simulink model "akh_rev_project"  (R2020b)
settings: Solver=ode45  StartTime=0.0  StopTime=10  FixedStep=Ts_Power  RelTol=1e-3  AbsTol=1e-2
InitFcn:
  | Fnom = 50;        % Hz
  | 
  | Fc = 27*Fnom;   % (Hz)
  | Ts_Power = 1/(Fc*100);
  | Ts_Control = Ts_Power*10;
values from neighbouring files (symbols this model uses):
  Ts = 1/fs    (= 1e-05)    [PE_46.m]    (also in disc_sim.m = 1; mass_spring_damper_model.m = 0.1)
undefined symbols (not defined in the file or in its folder): D1, D11, Delta, DiscIntNeverNeededParam, j, magnitude
libraries: powerlib x146, powerlib_meascontrol x90, simulink x2, re_lib x1
(part 1 of 8)
Description:
  | The 'Model  initialization function' defined in the
  | 
  | Model Properties automatically sets the sample time
  | 
  | Ts to 50e-6 s
settings Model: FPTRunName=Active  ExtModeTrigMode=oneshot  ExtModeArmWhenConnect=off  ExtModeAutoUpdateStatusClock=off  Creator=MathWorks  LastModifiedBy=Dhanush Wagle
settings SolverCC: AutoScaleAbsTol=off
settings DataIOCC: SaveFormat=StructureWithTime  SignalLoggingSaveFormat=ModelDataLogs  SaveTime=off  ReturnWorkspaceOutputs=off  SignalLoggingName=sigsOut
settings OptimizationCC: BlockReduction=off  BooleanDataType=off  ExpressionDepthLimit=2147483647  InitFltsAndDblsToZero=on  LifeSpan=inf
settings DebuggingCC: SaveWithParameterizedLinksMsg=none  UnderspecifiedInitializationDetection=Classic  MergeDetectMultiDrivingBlocksExec=none  CheckExecutionContextPreStartOutputMsg=on  CheckExecutionContextRuntimeOutputMsg=on  SignalResolutionControl=TryResolveAllWithWarning  MultiTaskDSMMsg=warning  MultiTaskCondExecSysMsg=none  FcnCallInpInsideContextMsg=warning  UnconnectedInputMsg=none  UnconnectedOutputMsg=none  UnconnectedLineMsg=none  StateNameClashWarn=warning  SFUnexpectedBacktrackingDiag=warning  SFNoUnconditionalDefaultTransitionDiag=warning  SFExecutionAtInitializationDiag=none  ArithmeticOperatorsInVariantConditions=warning
settings HardwareCC: ProdBitPerPointer=32  ProdBitPerSizeT=32  ProdBitPerPtrDiffT=32  ProdLargestAtomicFloat=None  ProdIntDivRoundTo=Undefined  ProdEndianess=Unspecified  ProdWordSize=32  ProdHWDeviceType=32-bit Generic  TargetHWDeviceType=32-bit Generic  ProdEqTarget=off
settings ModelReferenceCC: PropagateSignalLabelsOutOfModel=off
settings SFSimCC: SimUseLocalCustomCode=off  CustomCodeUndefinedFunction=UseInterfaceOnly
settings RTWCC: RTWUseLocalCustomCode=off
settings CodeAppCC: StateflowObjectComments=on
settings GRTTargetCC: TargetFcnLib=ansi_tfl_tmw.mat  TargetLangStandard=C89/C90 (ANSI)  CombineOutputUpdateFcns=off  GRTInterface=on
settings ConfigComp: CovMetricSettings=dw  CovSaveCumulativeToWorkspaceVar=on  CovSaveSingleToWorkspaceVar=on  CovExternalEMLEnable=off  CovSFcnEnable=off
settings SimscapeCC: SimscapeNormalizeSystem=off

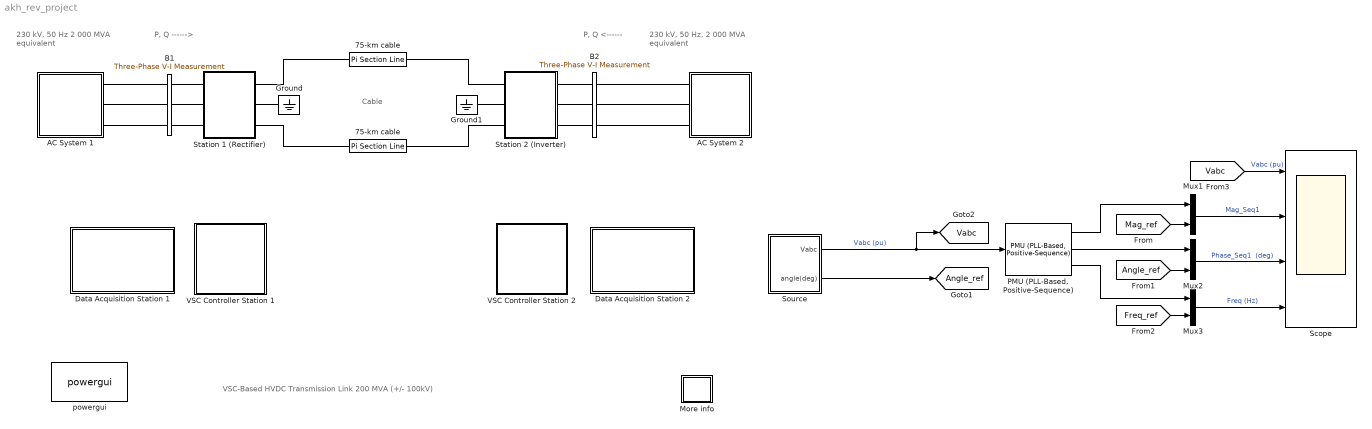
== system akh_rev_project ==
  note: VSC-Based HVDC Transmission Link 200 MVA (+/- 100kV)
  note: 230 kV, 50 Hz,
      | 2 000 MVA equivalent
  note: Cable
  note: P, Q
      | ------>
  note: P, Q
      | <------
  note: 230 kV, 50 Hz
      |  2 000 MVA equivalent
  75-km cable : powerlib/Elements/Pi Section Line  LConnTagsString=__new0  RConnTagsString=__new0  Phases=1  PiSections=2  Length=75  Frequency=Fnom  Resistance=1.3900e-002  Inductance=1.5900e-004  Capacitance=2.3100e-007  Measurements=None  Measurements2=None
      settings: AttributesFormatString=\n  SourceProductBaseCode=PS
  "75-km cable " : powerlib/Elements/Pi Section Line  LConnTagsString=__new0  RConnTagsString=__new0  Phases=1  PiSections=2  Length=75  Frequency=Fnom  Resistance=1.3900e-002  Inductance=1.5900e-004  Capacitance=2.3100e-007  Measurements=None  Measurements2=None
      settings: AttributesFormatString=\n  SourceProductBaseCode=PS
  AC System 1 : Subsystem
  AC System 2 : Subsystem
  B1 : powerlib/Measurements/Three-Phase V-I Measurement  VoltageMeasurement=phase-to-ground  SetLabelV=on  LabelV=Uabc_B1  Vpu=on  VpuLL=off  CurrentMeasurement=yes  SetLabelI=on  LabelI=Iabc_B1  Ipu=on  Pbase=200e6  Vbase=230e3  OutputType=Magnitude  PhasorSimulation=off  PSBequivalent=0
  B2 : powerlib/Measurements/Three-Phase V-I Measurement  VoltageMeasurement=phase-to-ground  SetLabelV=on  LabelV=Uabc_B2  Vpu=on  VpuLL=off  CurrentMeasurement=yes  SetLabelI=on  LabelI=Iabc_B2  Ipu=on  Pbase=200e6  Vbase=230e3  OutputType=Magnitude  PhasorSimulation=off  PSBequivalent=0
  Data Acquisition Station 1 : Subsystem
      mask Display: disp('Open this block\nto visualize\nrecorded signals')
  Data Acquisition Station 2 : Subsystem
      mask Display: disp('Open this block\nto visualize\nrecorded signals')
  Ground : powerlib/Elements/Ground  LConnTagsString=a
  Ground1 : powerlib/Elements/Ground  LConnTagsString=a
  More info : Subsystem
      settings: OpenFcn=showdemo(bdroot(gcb))
      mask Display: disp('?')
  Mux1 : Mux  Inputs=2
  Mux2 : Mux  Inputs=2
  Mux3 : Mux  Inputs=2
  "PMU (PLL-Based, Positive-Sequence)" : powerlib_meascontrol/Measurements/PMU (PLL-Based, Positive-Sequence)  nominalFrequency=60  samplingRate=64  reportingFactor=0.5
      settings: SourceProductBaseCode=PS
  Scope : Scope  NumInputPorts=4
  Source : Subsystem
  Station 1 (Rectifier) : Subsystem
  Station 2 (Inverter) : Subsystem
  VSC Controller Station 1 : Subsystem
      mask Display: disp('VSC\nPole Control')
  VSC Controller Station 2 : Subsystem
      mask Display: disp('VSC\nPole Control')
  powergui : powerlib/powergui  Priority=2  SimulationMode=Discrete  SampleTime=Ts_Power  frequency=60  Iterations=50  frequencyindice=60  Pbase=100e6  ErrMax=1e-4  UnitsV=kV  UnitsW=MW  buscounter=0  FunctionMessages=off  echomessages=off  EnableUseOfTLC=off  CurrentSourceSwitches=off  DisableSnubberDevices=off  DisableRonSwitches=off  DisableVfSwitches=off  DisplayEquations=off  AutomaticDiscreteSolvers=off  SolverType=Tustin/Backward Euler (TBE)  Interpol=off  ExternalGateDelay=off  methode=off  Ts=0  x0status=blocks  SPID=off  SwTol=0  HookPort=off  NonlinearTolerance=1e-4  nMaxIteration=100  ContinueOnMaxIteration=off  RestoreLinks=warning  ResistiveCurrentMeasurement=off  Frange=[0:2:500]  Ylog=off  Xlog=on  ShowGrid=off  save=off  variable=ZData  structure=res_fft  ZoomFFT=on  StartTime=1.5  cycles=2  DisplayStyle=1  fundamental=50  FreqAxis=off  MaxFrequency=3000  frequencyindicesteady=1  RmsSteady=1  display=off
  tag scope: Angle_ref=global, Vabc=global
  wires:
  [Mag_ref] -> Mux1/2
  Mux2/1 -> Scope/3  "Phase_Seq1  (deg)"
  Source/2(angle(deg)) -> [Angle_ref]
  "PMU (PLL-Based, Positive-Sequence)"/2 -> Mux2/1
  "PMU (PLL-Based, Positive-Sequence)"/3 -> Mux3/1
  [Vabc] -> Scope/1  "Vabc (pu)"
  [Angle_ref] -> Mux2/2
  [Freq_ref] -> Mux3/2
  Mux3/1 -> Scope/4  "Freq (Hz)"
  Mux1/1 -> Scope/2  "Mag_Seq1"
  "PMU (PLL-Based, Positive-Sequence)"/1 -> Mux1/1
  Source/1(Vabc) -> [Vabc], "PMU (PLL-Based, Positive-Sequence)"/1  "Vabc (pu)"
  connections:
  Station 1 (Rectifier)/LConn1 -- B1/RConn1
  B1/RConn2 -- Station 1 (Rectifier)/LConn2
  Station 1 (Rectifier)/LConn3 -- B1/RConn3
  "75-km cable "/LConn1 -- Station 1 (Rectifier)/RConn3
  75-km cable/RConn1 -- Station 2 (Inverter)/RConn1
  "75-km cable "/RConn1 -- Station 2 (Inverter)/RConn3
  B2/LConn1 -- AC System 2/RConn1
  Station 2 (Inverter)/LConn1 -- B2/RConn1
  Station 2 (Inverter)/LConn2 -- B2/RConn2
  Station 2 (Inverter)/LConn3 -- B2/RConn3
  B2/LConn2 -- AC System 2/RConn2
  B2/LConn3 -- AC System 2/RConn3
  Ground/LConn1 -- Station 1 (Rectifier)/RConn2
  Ground1/LConn1 -- Station 2 (Inverter)/RConn2
  AC System 1/RConn1 -- B1/LConn1
  AC System 1/RConn2 -- B1/LConn2
  AC System 1/RConn3 -- B1/LConn3
  Station 1 (Rectifier)/RConn1 -- 75-km cable/LConn1

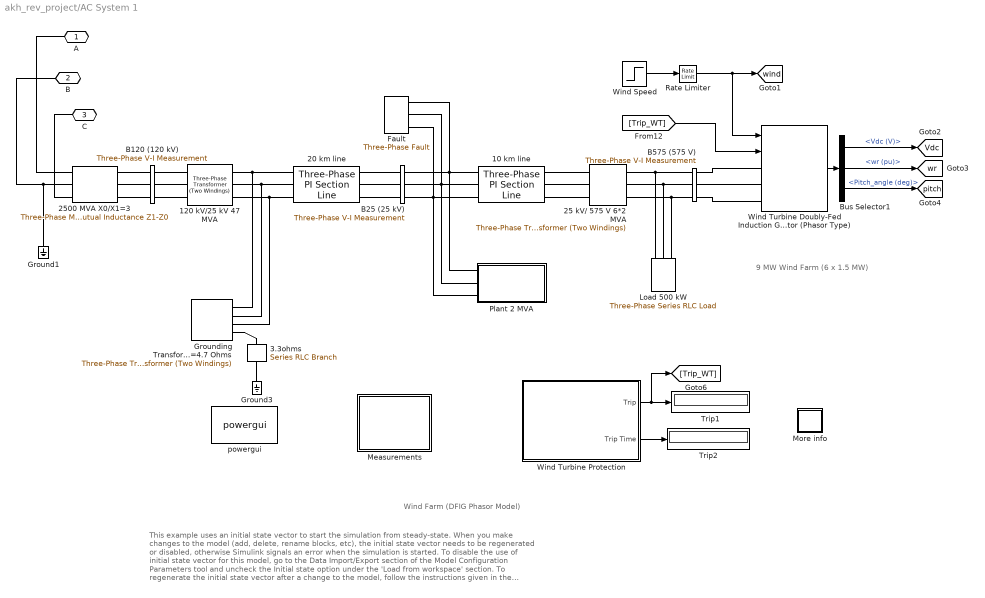
== system akh_rev_project/AC System 1 ==
  note: This example uses an initial state vector to start the simulation from steady-state. When you make changes to the model (add, delete, rename blocks, etc),
      | the initial state vector needs to be regenerated or disabled, otherwise Simulink signals an error when the simulation is started.
      | To disable the use of initial state vector for this model, go to the Data Import/Export section of the Model Configuration Parameters tool and uncheck the
      | Initial state option under the 'Load from workspace' section.
      | To regenerate the initial state vector after a change to the model, follow the instructions given in the initialization file for this model.
      | Type open('init_power_wind_dfig') at the matlab prompt to view this file.
  note: 9 MW Wind Farm
      | (6 x 1.5 MW)
  note: Wind Farm (DFIG Phasor Model)
  10 km line : powerlib/Elements/Three-Phase PI Section Line  LConnTagsString=a|b|c  RConnTagsString=A|B|C  Length=10  Frequency=60  Resistances=[0.1153 0.413]  Inductances=[1.05e-3 3.32e-3]  Capacitances=[11.33e-009 5.01e-009]
  120 kV/25 kV 47 MVA : powerlib/Elements/Three-Phase Transformer (Two Windings)  Winding1Connection=Yg  Winding2Connection=Delta (D1)  CoreType=Three single-phase transformers  SetSaturation=off  Hysteresis=off  DataFile='basic_model'  SetInitialFlux=off  Measurements=None  UNITS=pu  NominalPower=[47e6 60 ]  Winding1="[ 120e3  0.08/30   0.08 ]"  Winding2="[ 25e3  0.08/30  0.08]"  Rm=500  Lm=500  L0=0.5  Saturation="[ 0,0  ;  0.005,1.2  ;  1.0,1.4 ]"  InitialFluxes=[ 0.8 , -0.8 , 0.7 ]  BreakLoop=off  DiscreteSolver=Trapezoidal iterative  DataType=off  TransfoNumber=0
  20 km line : powerlib/Elements/Three-Phase PI Section Line  LConnTagsString=a|b|c  RConnTagsString=A|B|C  Length=20  Frequency=60  Resistances=[0.1153 0.413]  Inductances=[1.05e-3 3.32e-3]  Capacitances=[11.33e-009 5.01e-009]
  25 kV/ 575 V 6*2 MVA : powerlib/Elements/Three-Phase Transformer (Two Windings)  Winding1Connection=Yg  Winding2Connection=Delta (D1)  CoreType=Three single-phase transformers  SetSaturation=off  Hysteresis=off  DataFile='hysteresis'  SetInitialFlux=off  Measurements=None  UNITS=pu  NominalPower="[2e6*6  60]"  Winding1=[25e3 , 0.025/30 , 0.025]  Winding2=[ 575, 0.025/30 , 0.025]  Rm=500  Lm=inf  L0=0.5  Saturation=[ 0,0 ; 0.0024,1.2 ; 1.0,1.52 ]  InitialFluxes=[ 0.8 , -0.8 , 0.7 ]  BreakLoop=off  DiscreteSolver=Trapezoidal iterative  DataType=off  TransfoNumber=0
  2500 MVA X0/X1=3 : powerlib/Elements/Three-Phase Mutual Inductance Z1-Z0  LConnTagsString=a|b|c  RConnTagsString=A|B|C  PositiveSequence="[0.1  1.0/(2*pi*60)] *120e3^2/2500e6"  ZeroSequence="[0.3  3.0/(2*pi*60)] *120e3^2/2500e6"
      settings: SourceProductBaseCode=PS
  "3.3ohms " : powerlib/Elements/Series RLC Branch  LConnTagsString=__new0  RConnTagsString=__new0  BranchType=R  Resistance=3.3  Inductance=1.0  SetiL0=off  InitialCurrent=0  Capacitance=1.0  Setx0=off  InitialVoltage=0  Measurements=None
  B120 (120 kV) : powerlib/Measurements/Three-Phase V-I Measurement  VoltageMeasurement=phase-to-ground  SetLabelV=on  LabelV=Vabc_B120  Vpu=on  VpuLL=off  CurrentMeasurement=no  SetLabelI=on  LabelI=Iabc_B120  Ipu=off  Pbase=100e6  Vbase=120e3  OutputType=Complex  PhasorSimulation=on  PSBequivalent=0
  B25 (25 kV) : powerlib/Measurements/Three-Phase V-I Measurement  VoltageMeasurement=phase-to-ground  SetLabelV=on  LabelV=Vabc_B25  Vpu=on  VpuLL=off  CurrentMeasurement=yes  SetLabelI=on  LabelI=Iabc_B25  Ipu=on  Pbase=10e6  Vbase=25e3  OutputType=Complex  PhasorSimulation=on  PSBequivalent=0
  B575 (575 V) : powerlib/Measurements/Three-Phase V-I Measurement  VoltageMeasurement=phase-to-ground  SetLabelV=on  LabelV=Vabc_B575  Vpu=on  VpuLL=off  CurrentMeasurement=yes  SetLabelI=on  LabelI=Iabc_B575  Ipu=on  Pbase=6*1.5e6/0.9  Vbase=575  OutputType=Complex  PhasorSimulation=on  PSBequivalent=0
  Bus Selector1 : BusSelector  OutputSignals=Vdc (V),wr (pu),Pitch_angle (deg)
  Fault : powerlib/Elements/Three-Phase Fault  InitialStates=0  FaultA=off  FaultB=off  FaultC=off  GroundFault=on  SwitchTimes=[ 5 5+9/60]  External=off  SwitchStatus=NaN  FaultResistance=1e-3  GroundResistance=1e-3  SnubberResistance=1e4  SnubberCapacitance=inf  Measurements=None
  Ground1 : powerlib/Elements/Ground  LConnTagsString=a
  Ground3 : powerlib/Elements/Ground  LConnTagsString=a
  Grounding Transformer X0=4.7 Ohms : powerlib/Elements/Three-Phase Transformer (Two Windings)  Winding1Connection=Yn  Winding2Connection=Delta (D11)  CoreType=Three single-phase transformers  SetSaturation=off  Hysteresis=off  DataFile='basic_model'  SetInitialFlux=off  Measurements=None  UNITS=pu  NominalPower=[100e6 60]  Winding1="[ 25e3  4.7/(25e3^2/100e6)/30    4.7/(25e3^2/100e6)]"  Winding2="[ 25e3  1e-6  0]"  Rm=500  Lm=500  L0=0.5  Saturation="[ 0,0  ;  0.005,1.2  ;  1.0,1.4 ]"  InitialFluxes=[ 0.8 , -0.8 , 0.7 ]  BreakLoop=off  DiscreteSolver=Trapezoidal iterative  DataType=off  TransfoNumber=0
  Load 500 kW : powerlib/Elements/Three-Phase Series RLC Load  LConnTagsString=A|B|C  Configuration=Y (grounded)  NominalVoltage=575  Vabc=[1e3 1e3 1e3]  Vabcp=[1e3 1e3 1e3]  NominalFrequency=60  UnbalancedPower=off  ActivePower=500e3  InductivePower=0  CapacitivePower=0  Pabc=[10e3 9e3 11e3]  QLabc=[100 90 110]  QCabc=[100 90 110]  Pabcp=[10e3 9e3 11e3]  QLabcp=[100 90 110]  QCabcp=[100 90 110]  Measurements=None  LoadType=constant Z
  Measurements : Subsystem
  More info : Subsystem
      settings: OpenFcn=showdemo(bdroot(gcb))
      mask Display: disp('?')
  Plant 2 MVA : Subsystem
  Rate Limiter : RateLimiter
  Trip1 : Display
  Trip2 : Display
  Wind Speed : Step  Time=5  Before=8  After=14  SampleTime=0
  Wind Turbine Doubly-Fed Induction Generator (Phasor Type) : re_lib/Wind Generation/Wind Turbine Doubly-Fed Induction Generator (Phasor Type)  ExternalTm=off  nom=[6*1.5e6/0.9 575 60]  sta=[ 0.00706 0.171]  rot=[ 0.005 0.156]  Lm=2.9  mec=[5.04 0.01 3]  init=[0.2 0 0 0 0 0]  speed_power=[0 0; 0.24 0.007; 0.36 0.024; 0.6 0.112; 0.96 0.46; 1.2 0.898; 1.5 0.898]  Pmec=6*1.5e6  speed_ABCD=[0.7 0.71 1.2 1.21]  power_C=0.73  wind_point_C=12  pitch_gain=500  pitch_max=45  pitch_rate=2  Pmax=0.5  Lchoke=[0.15 0.15/100]  init_inductor=[0 90]  Vdc_nom=1200  capacitor=6*10000e-6  ControlVQ=Voltage regulation  Vref=1.0  ExternalVref=off  Qref=0  ExternalQref=off  Iq_ref=0  ExternalIqref=off  Kpi_volt_reg=[1.25 300]  Xs=0.02  Kpi_Q=[0.05 5]  Kpi_power_reg=[1 100]  Kpi_dc_reg=[0.002 0.05]  Kpi_grid_side_cur_reg=[1 100]  Kpi_rotor_side_cur_reg=[0.3 8]  V_slew_rate=100  Q_slew_rate=100  power_slew_rate=1  current_slew_rate=200
      settings: SourceProductBaseCode=PS
  Wind Turbine Protection : Subsystem
      mask Display: disp('Wind\nTurbine\nProtection')
  powergui : powerlib/powergui  Priority=2  SimulationMode=Phasor  SampleTime=0  frequency=60  Iterations=50  frequencyindice=60  Pbase=100e6  ErrMax=1e-4  UnitsV=kV  UnitsW=MW  buscounter=0  FunctionMessages=off  echomessages=off  EnableUseOfTLC=off  CurrentSourceSwitches=off  DisableSnubberDevices=off  DisableRonSwitches=off  DisableVfSwitches=off  DisplayEquations=off  AutomaticDiscreteSolvers=off  SolverType=Tustin  Interpol=off  ExternalGateDelay=off  methode=off  Ts=0  x0status=blocks  SPID=off  SwTol=0  HookPort=off  NonlinearTolerance=1e-4  nMaxIteration=100  ContinueOnMaxIteration=off  RestoreLinks=warning  ResistiveCurrentMeasurement=off  Frange=[0:2:500]  Ylog=off  Xlog=off  ShowGrid=off  save=off  variable=ZData  structure=0  ZoomFFT=on  StartTime=0.0  cycles=1  DisplayStyle=1  fundamental=60  FreqAxis=off  MaxFrequency=1000  frequencyindicesteady=1  RmsSteady=1  display=off
  A : PMIOPort  Side=Right
  B : PMIOPort  Port=2  Side=Right
  C : PMIOPort  Port=3  Side=Right
  tag scope: Vdc=global, pitch=global, wind=global, wr=global
  wires:
  [Trip_WT] -> Wind Turbine Doubly-Fed Induction Generator (Phasor Type)/2
  Bus Selector1/3 -> [pitch]  "<Pitch_angle (deg)>"
  Wind Turbine Doubly-Fed Induction Generator (Phasor Type)/1 -> Bus Selector1/1
  Bus Selector1/1 -> [Vdc]  "<Vdc (V)>"
  Wind Turbine Protection/2(Trip Time) -> Trip2/1
  Bus Selector1/2 -> [wr]  "<wr (pu)>"
  Rate Limiter/1 -> Wind Turbine Doubly-Fed Induction Generator (Phasor Type)/1, [wind]
  Wind Speed/1 -> Rate Limiter/1
  Wind Turbine Protection/1(Trip) -> [Trip_WT], Trip1/1
  connections:
  B575 (575 V)/LConn3 -- Load 500 kW/LConn3 -- 25 kV/ 575 V 6*2 MVA/RConn3
  10 km line/LConn1 -- Fault/LConn1 -- B25 (25 kV)/RConn1 -- Plant 2 MVA/LConn1
  B575 (575 V)/LConn2 -- Load 500 kW/LConn2 -- 25 kV/ 575 V 6*2 MVA/RConn2
  10 km line/LConn2 -- Fault/LConn2 -- B25 (25 kV)/RConn2 -- Plant 2 MVA/LConn2
  10 km line/LConn3 -- Fault/LConn3 -- B25 (25 kV)/RConn3 -- Plant 2 MVA/LConn3
  Grounding Transformer X0=4.7 Ohms/LConn1 -- 120 kV/25 kV 47 MVA/RConn1 -- 20 km line/LConn1
  B575 (575 V)/LConn1 -- Load 500 kW/LConn1 -- 25 kV/ 575 V 6*2 MVA/RConn1
  Grounding Transformer X0=4.7 Ohms/LConn3 -- 120 kV/25 kV 47 MVA/RConn3 -- 20 km line/LConn3
  Grounding Transformer X0=4.7 Ohms/LConn2 -- 120 kV/25 kV 47 MVA/RConn2 -- 20 km line/LConn2
  C/RConn1 -- 2500 MVA X0/X1=3/LConn3
  B25 (25 kV)/LConn1 -- 20 km line/RConn1
  10 km line/RConn2 -- 25 kV/ 575 V 6*2 MVA/LConn2
  B575 (575 V)/RConn1 -- Wind Turbine Doubly-Fed Induction Generator (Phasor Type)/LConn1
  B575 (575 V)/RConn2 -- Wind Turbine Doubly-Fed Induction Generator (Phasor Type)/LConn2
  B120 (120 kV)/RConn1 -- 120 kV/25 kV 47 MVA/LConn1
  10 km line/RConn3 -- 25 kV/ 575 V 6*2 MVA/LConn3
  B120 (120 kV)/RConn2 -- 120 kV/25 kV 47 MVA/LConn2
  10 km line/RConn1 -- 25 kV/ 575 V 6*2 MVA/LConn1
  B120 (120 kV)/LConn3 -- 2500 MVA X0/X1=3/RConn3
  A/RConn1 -- 2500 MVA X0/X1=3/LConn1
  B575 (575 V)/RConn3 -- Wind Turbine Doubly-Fed Induction Generator (Phasor Type)/LConn3
  20 km line/RConn2 -- B25 (25 kV)/LConn2
  "3.3ohms "/RConn1 -- Ground3/LConn1
  B120 (120 kV)/RConn3 -- 120 kV/25 kV 47 MVA/LConn3
  20 km line/RConn3 -- B25 (25 kV)/LConn3
  B/RConn1 -- Ground1/LConn1 -- 2500 MVA X0/X1=3/LConn2
  Grounding Transformer X0=4.7 Ohms/LConn4 -- "3.3ohms "/LConn1
  B120 (120 kV)/LConn2 -- 2500 MVA X0/X1=3/RConn2
  B120 (120 kV)/LConn1 -- 2500 MVA X0/X1=3/RConn1

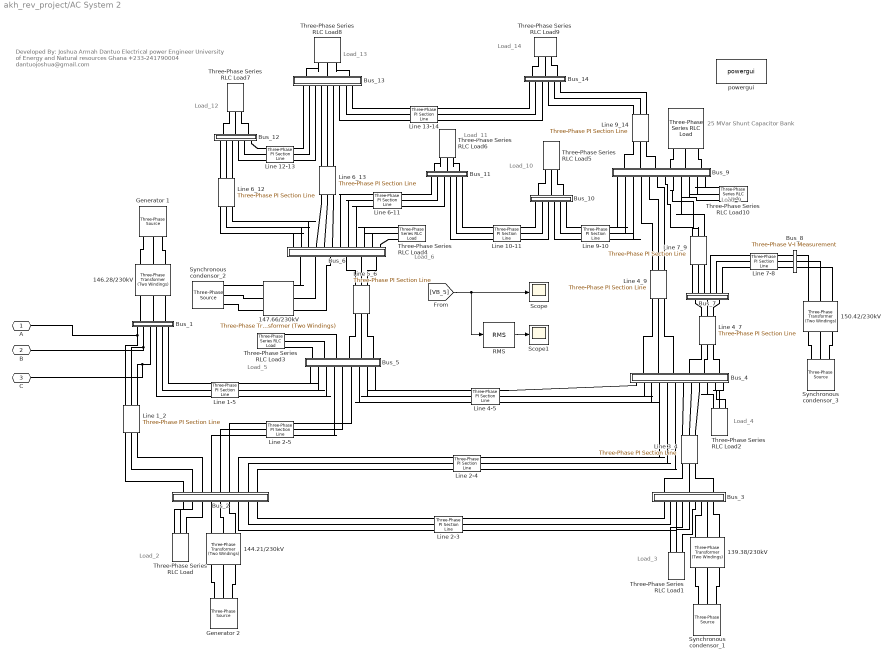
== system akh_rev_project/AC System 2 ==
  note: Load_14
  note: Load_4
  note: Developed By:
      | Joshua Armah Dantuo
      | Electrical power Engineer
      | University of Energy and Natural resources
      | Ghana
      | +233-241790004
      | dantuojoshua@gmail.com
  note: Load_3
  note: Load_5
  note: Load_12
  note: Load_10
  note: Load_9
  note: 25 MVar Shunt
      | Capacitor Bank
  note: Load_11
  note: Load_2
  note: Load_6
  note: Load_13
  " " : powerlib/Elements/Three-Phase Series RLC Load  LConnTagsString=A|B|C  Configuration=Y (grounded)  NominalVoltage=230e3  Vabc=[1e3 1e3 1e3]  Vabcp=[1e3 1e3 1e3]  NominalFrequency=60  UnbalancedPower=off  ActivePower=0  InductivePower=0  CapacitivePower=25e6  Pabc=[10e3 9e3 11e3]  QLabc=[100 90 110]  QCabc=[100 90 110]  Pabcp=[10e3 9e3 11e3]  QLabcp=[100 90 110]  QCabcp=[100 90 110]  Measurements=None  LoadType=constant Z
  139.38/230kV : powerlib/Elements/Three-Phase Transformer (Two Windings)  Winding1Connection=Yg  Winding2Connection=Yg  CoreType=Three single-phase transformers  SetSaturation=off  Hysteresis=off  DataFile='hysteresis'  SetInitialFlux=off  Measurements=None  UNITS=pu  NominalPower=[ 120e6 , 60 ]  Winding1=[139.38e3 , 0.002 , 0.08 ]  Winding2=[ 230e3 , 0.002 , 0.08 ]  Rm=500  Lm=500  L0=0.5  Saturation=[ 0,0 ; 0.0024,1.2 ; 1.0,1.52 ]  InitialFluxes=[ 0.8 , -0.8 , 0.7 ]  BreakLoop=off  DiscreteSolver=Trapezoidal iterative  DataType=off  TransfoNumber=1
  144.21/230kV : powerlib/Elements/Three-Phase Transformer (Two Windings)  Winding1Connection=Yg  Winding2Connection=Yg  CoreType=Three single-phase transformers  SetSaturation=off  Hysteresis=off  DataFile='hysteresis'  SetInitialFlux=off  Measurements=None  UNITS=pu  NominalPower=[ 120e6 , 60 ]  Winding1=[144.21e3 , 0.002 , 0.08 ]  Winding2=[ 230e3 , 0.002 , 0.08 ]  Rm=500  Lm=500  L0=0.5  Saturation=[ 0,0 ; 0.0024,1.2 ; 1.0,1.52 ]  InitialFluxes=[ 0.8 , -0.8 , 0.7 ]  BreakLoop=off  DiscreteSolver=Trapezoidal iterative  DataType=off  TransfoNumber=1
  146.28/230kV : powerlib/Elements/Three-Phase Transformer (Two Windings)  Winding1Connection=Yg  Winding2Connection=Yg  CoreType=Three single-phase transformers  SetSaturation=off  Hysteresis=off  DataFile='hysteresis'  SetInitialFlux=off  Measurements=None  UNITS=pu  NominalPower=[ 120e6 , 60 ]  Winding1=[146.28e3 , 0.002 , 0.08 ]  Winding2=[ 230e3 , 0.002 , 0.08 ]  Rm=500  Lm=500  L0=0.5  Saturation=[ 0,0 ; 0.0024,1.2 ; 1.0,1.52 ]  InitialFluxes=[ 0.8 , -0.8 , 0.7 ]  BreakLoop=off  DiscreteSolver=Trapezoidal iterative  DataType=off  TransfoNumber=1
  147.66/230kV : powerlib/Elements/Three-Phase Transformer (Two Windings)  Winding1Connection=Yg  Winding2Connection=Yg  CoreType=Three single-phase transformers  SetSaturation=off  Hysteresis=off  DataFile='hysteresis'  SetInitialFlux=off  Measurements=None  UNITS=pu  NominalPower=[ 120e6 , 60 ]  Winding1=[147.66e3 , 0.002 , 0.08 ]  Winding2=[ 230e3 , 0.002 , 0.08 ]  Rm=500  Lm=500  L0=0.5  Saturation=[ 0,0 ; 0.0024,1.2 ; 1.0,1.52 ]  InitialFluxes=[ 0.8 , -0.8 , 0.7 ]  BreakLoop=off  DiscreteSolver=Trapezoidal iterative  DataType=off  TransfoNumber=1
  150.42/230kV : powerlib/Elements/Three-Phase Transformer (Two Windings)  Winding1Connection=Yg  Winding2Connection=Yg  CoreType=Three single-phase transformers  SetSaturation=off  Hysteresis=off  DataFile='hysteresis'  SetInitialFlux=off  Measurements=None  UNITS=pu  NominalPower=[ 120e6 , 60 ]  Winding1=[150.42e3 , 0.002 , 0.08 ]  Winding2=[ 230e3 , 0.002 , 0.08 ]  Rm=500  Lm=500  L0=0.5  Saturation=[ 0,0 ; 0.0024,1.2 ; 1.0,1.52 ]  InitialFluxes=[ 0.8 , -0.8 , 0.7 ]  BreakLoop=off  DiscreteSolver=Trapezoidal iterative  DataType=off  TransfoNumber=1
  Bus_1 : Subsystem
  Bus_10 : Subsystem
  Bus_11 : Subsystem
  Bus_12 : Subsystem
  Bus_13 : Subsystem
  Bus_14 : Subsystem
  Bus_2 : Subsystem
  Bus_3 : Subsystem
  Bus_4 : Subsystem
  Bus_5 : Subsystem
  Bus_6 : Subsystem
  Bus_7 : Subsystem
  Bus_8 : powerlib/Measurements/Three-Phase V-I Measurement  VoltageMeasurement=phase-to-phase  SetLabelV=on  LabelV=VB_8  Vpu=off  VpuLL=off  CurrentMeasurement=yes  SetLabelI=on  LabelI=IB_8  Ipu=off  Pbase=100e6  Vbase=500e3  OutputType=Complex  PhasorSimulation=off  PSBequivalent=0
  Bus_9 : Subsystem
  Generator 1 : powerlib/Electrical Sources/Three-Phase Source  InternalConnection=Yg  VoltagePhases=off  Voltage=(146280)*1.03071  PhaseAngle=3.7708  Voltage_phases=[25e3 25e3 25e3]/sqrt(3)  PhaseAngles_phases=[0 -120 +120]  Frequency=60  NonIdealSource=on  SpecifyImpedance=off  Resistance=0.8929  Inductance=16.58e-3  ShortCircuitLevel=100e6  BaseVoltage=146.28e3  XRratio=7  BusType=swing  Pref=163e6  Qref=0  Prefabc=[10e3, 10e3, 10e3]  Qrefabc=[0, 0, 0]  Qmin=-inf  Qmax=inf
  Generator 2 : powerlib/Electrical Sources/Three-Phase Source  InternalConnection=Yg  VoltagePhases=off  Voltage=(144210)*1.01655  PhaseAngle=-15.8323  Voltage_phases=[25e3 25e3 25e3]/sqrt(3)  PhaseAngles_phases=[0 -120 +120]  Frequency=60  NonIdealSource=on  SpecifyImpedance=off  Resistance=0.8929  Inductance=16.58e-3  ShortCircuitLevel=100e6  BaseVoltage=144.21e3  XRratio=7  BusType=PV  Pref=90e6  Qref=0  Prefabc=[10e3, 10e3, 10e3]  Qrefabc=[0, 0, 0]  Qmin=-inf  Qmax=inf
  Line 1-5 : powerlib/Elements/Three-Phase PI Section Line  LConnTagsString=a|b|c  RConnTagsString=A|B|C  Length=78.64  Frequency=60  Resistances=[ 0.3029 0.9086]  Inductances=[ 0.0033 0.0099]  Capacitances=[3.35e-9 1.01e-8]
  Line 10-11 : powerlib/Elements/Three-Phase PI Section Line  LConnTagsString=a|b|c  RConnTagsString=A|B|C  Length=4.93  Frequency=60  Resistances=[ 0.3667 1.1002]  Inductances=[ 0.0023 0.0068]  Capacitances=[1.22e-11 3.66e-11]
  Line 12-13 : powerlib/Elements/Three-Phase PI Section Line  LConnTagsString=a|b|c  RConnTagsString=A|B|C  Length=5.03  Frequency=60  Resistances=[ 0.9679 2.9038]  Inductances=[ 0.0023 0.0070]  Capacitances=[1.20e-11 3.59e-11]
  Line 13-14 : powerlib/Elements/Three-Phase PI Section Line  LConnTagsString=a|b|c  RConnTagsString=A|B|C  Length=6.64  Frequency=60  Resistances=[ 0.5676 1.7027]  Inductances=[ 0.0031 0.0092]  Capacitances=[9.06e-12 2.72e-11]
  Line 1_2 : powerlib/Elements/Three-Phase PI Section Line  LConnTagsString=a|b|c  RConnTagsString=A|B|C  Length=44.47  Frequency=60  Resistances=[ 0.1921 0.5763]  Inductances=[ 0.0016 0.0047]  Capacitances=[7.14e-9 2.14e-8]
  Line 2-3 : powerlib/Elements/Three-Phase PI Section Line  LConnTagsString=a|b|c  RConnTagsString=A|B|C  Length=68.47  Frequency=60  Resistances=[ 0.3026 0.9077]  Inductances=[ 0.0034 0.0101]  Capacitances=[3.29e-9 9.86e-8]
  Line 2-4 : powerlib/Elements/Three-Phase PI Section Line  LConnTagsString=a|b|c  RConnTagsString=A|B|C  Length=74.11  Frequency=60  Resistances=[ 0.3457 1.0370]  Inductances=[ 0.0028 0.0083]  Capacitances=[3.99e-9 1.20e-8]
  Line 2-5 : powerlib/Elements/Three-Phase PI Section Line  LConnTagsString=a|b|c  RConnTagsString=A|B|C  Length=61.18  Frequency=60  Resistances=[ 0.4104 1.2311]  Inductances=[ 0.0033 0.0100]  Capacitances=[3.34e-9 1.0e-8]
  Line 3_4 : powerlib/Elements/Three-Phase PI Section Line  LConnTagsString=a|b|c  RConnTagsString=A|B|C  Length=61.21  Frequency=60  Resistances=[ 0.4826 1.4479]  Inductances=[ 0.0033 0.0098]  Capacitances=[3.4e-9 1.02e-8]
  Line 4-5 : powerlib/Elements/Three-Phase PI Section Line  LConnTagsString=a|b|c  RConnTagsString=A|B|C  Length=18.47  Frequency=60  Resistances=[ 0.3186 0.9558]  Inductances=[ 0.0027 0.0080]  Capacitances=[4.17e-9 1.25e-8]
  Line 4_7 : powerlib/Elements/Three-Phase PI Section Line  LConnTagsString=a|b|c  RConnTagsString=A|B|C  Length=5.15  Frequency=60  Resistances=[ 0.0001 0.0003]  Inductances=[ 0.0475 0.1425]  Capacitances=[2.34e-10 7.02e-10]
  Line 4_9 : powerlib/Elements/Three-Phase PI Section Line  LConnTagsString=a|b|c  RConnTagsString=A|B|C  Length=8.39  Frequency=60  Resistances=[ 0.0001 0.0003]  Inductances=[ 0.0775 0.2325]  Capacitances=[1.43e-10 4.3e-10]
  Line 5_6 : powerlib/Elements/Three-Phase PI Section Line  LConnTagsString=a|b|c  RConnTagsString=A|B|C  Length=5.65  Frequency=60  Resistances=[ 0.0001 0.0003]  Inductances=[ 0.0522 0.1565]  Capacitances=[2.13e-10 6.39e-10]
  Line 6-11 : powerlib/Elements/Three-Phase PI Section Line  LConnTagsString=a|b|c  RConnTagsString=A|B|C  Length=5.02  Frequency=60  Resistances=[ 0.4172 1.2515]  Inductances=[ 0.0023 0.0070]  Capacitances=[1.20e-11 3.60e-11]
  Line 6_12 : powerlib/Elements/Three-Phase PI Section Line  LConnTagsString=a|b|c  RConnTagsString=A|B|C  Length=5.69  Frequency=60  Resistances=[ 0.4760 1.4281]  Inductances=[ 0.0026 0.0079]  Capacitances=[1.06e-11 3.17e-11]
  Line 6_13 : powerlib/Elements/Three-Phase PI Section Line  LConnTagsString=a|b|c  RConnTagsString=A|B|C  Length=4.06  Frequency=60  Resistances=[ 0.3590 1.0770]  Inductances=[ 0.0019 0.0056]  Capacitances=[1.48e-11 4.44e-11]
  Line 7-8 : powerlib/Elements/Three-Phase PI Section Line  LConnTagsString=a|b|c  RConnTagsString=A|B|C  Length=4.72  Frequency=60  Resistances=[ 0.0005 0.0014]  Inductances=[ 0.0022 0.0065]  Capacitances=[ 1.27e-11 3.82e-11]
  Line 7_9 : powerlib/Elements/Three-Phase PI Section Line  LConnTagsString=a|b|c  RConnTagsString=A|B|C  Length=3.73  Frequency=60  Resistances=[ 0.0006 0.0018]  Inductances=[ 0.0017 0.0052]  Capacitances=[ 1.61e-11 4.84e-11]
  Line 9-10 : powerlib/Elements/Three-Phase PI Section Line  LConnTagsString=a|b|c  RConnTagsString=A|B|C  Length=3.27  Frequency=60  Resistances=[ 0.2144 0.6431]  Inductances=[ 0.0015 0.0045]  Capacitances=[1.84e-11 5.52e-11]
  Line 9_14 : powerlib/Elements/Three-Phase PI Section Line  LConnTagsString=a|b|c  RConnTagsString=A|B|C  Length=5.85  Frequency=60  Resistances=[ 0.4788 1.4365]  Inductances=[ 0.0027 0.0081]  Capacitances=[1.03e-11 3.08e-11]
  RMS : powerlib_meascontrol/Measurements/RMS  TrueRMS=on  Freq=60  RMSInit=120  Ts=0
  Scope : Scope
  Scope1 : Scope
  Synchronous condensor_1 : powerlib/Electrical Sources/Three-Phase Source  InternalConnection=Yg  VoltagePhases=off  Voltage=(139380)*1.01137  PhaseAngle=-34.48  Voltage_phases=[25e3 25e3 25e3]/sqrt(3)  PhaseAngles_phases=[0 -120 +120]  Frequency=60  NonIdealSource=on  SpecifyImpedance=off  Resistance=0.8929  Inductance=16.58e-3  ShortCircuitLevel=100e6  BaseVoltage=139.38e3  XRratio=7  BusType=PQ  Pref=0  Qref=50.096e6  Prefabc=[10e3, 10e3, 10e3]  Qrefabc=[0, 0, 0]  Qmin=-inf  Qmax=inf
  Synchronous condensor_2 : powerlib/Electrical Sources/Three-Phase Source  InternalConnection=Yg  VoltagePhases=off  Voltage=(147660)*0.984306  PhaseAngle=-36.2022  Voltage_phases=[25e3 25e3 25e3]/sqrt(3)  PhaseAngles_phases=[0 -120 +120]  Frequency=60  NonIdealSource=on  SpecifyImpedance=off  Resistance=0.8929  Inductance=16.58e-3  ShortCircuitLevel=100e6  BaseVoltage=147.66e3  XRratio=7  BusType=PQ  Pref=0  Qref=25.276e6  Prefabc=[10e3, 10e3, 10e3]  Qrefabc=[0, 0, 0]  Qmin=-inf  Qmax=inf
  Synchronous condensor_3 : powerlib/Electrical Sources/Three-Phase Source  InternalConnection=Yg  VoltagePhases=off  Voltage=(150420)*0.995122  PhaseAngle=-36.1424  Voltage_phases=[25e3 25e3 25e3]/sqrt(3)  PhaseAngles_phases=[0 -120 +120]  Frequency=60  NonIdealSource=on  SpecifyImpedance=off  Resistance=0.8929  Inductance=16.58e-3  ShortCircuitLevel=100e6  BaseVoltage=150.42e3  XRratio=7  BusType=PQ  Pref=0  Qref=30.144e6  Prefabc=[10e3, 10e3, 10e3]  Qrefabc=[0, 0, 0]  Qmin=-inf  Qmax=inf
  Three-Phase Series RLC Load : powerlib/Elements/Three-Phase Series RLC Load  LConnTagsString=A|B|C  Configuration=Y (grounded)  NominalVoltage=(230000)*0.949726  Vabc=[1e3 1e3 1e3]  Vabcp=[1e3 1e3 1e3]  NominalFrequency=60  UnbalancedPower=off  ActivePower=26.04e6  InductivePower=15.24e6  CapacitivePower=0  Pabc=[10e3 9e3 11e3]  QLabc=[100 90 110]  QCabc=[100 90 110]  Pabcp=[10e3 9e3 11e3]  QLabcp=[100 90 110]  QCabcp=[100 90 110]  Measurements=None  LoadType=constant PQ
  Three-Phase Series RLC Load1 : powerlib/Elements/Three-Phase Series RLC Load  LConnTagsString=A|B|C  Configuration=Y (grounded)  NominalVoltage=(230000)*0.92821  Vabc=[1e3 1e3 1e3]  Vabcp=[1e3 1e3 1e3]  NominalFrequency=60  UnbalancedPower=off  ActivePower=113.04e6  InductivePower=22.8e6  CapacitivePower=0  Pabc=[10e3 9e3 11e3]  QLabc=[100 90 110]  QCabc=[100 90 110]  Pabcp=[10e3 9e3 11e3]  QLabcp=[100 90 110]  QCabcp=[100 90 110]  Measurements=None  LoadType=constant PQ
  Three-Phase Series RLC Load10 : powerlib/Elements/Three-Phase Series RLC Load  LConnTagsString=A|B|C  Configuration=Y (grounded)  NominalVoltage=(230000)*0.942986  Vabc=[1e3 1e3 1e3]  Vabcp=[1e3 1e3 1e3]  NominalFrequency=60  UnbalancedPower=off  ActivePower=35.4e6  InductivePower=19.92e6  CapacitivePower=0  Pabc=[10e3 9e3 11e3]  QLabc=[100 90 110]  QCabc=[100 90 110]  Pabcp=[10e3 9e3 11e3]  QLabcp=[100 90 110]  QCabcp=[100 90 110]  Measurements=None  LoadType=constant PQ
  Three-Phase Series RLC Load2 : powerlib/Elements/Three-Phase Series RLC Load  LConnTagsString=A|B|C  Configuration=Y (grounded)  NominalVoltage=(230000)*0.927953  Vabc=[1e3 1e3 1e3]  Vabcp=[1e3 1e3 1e3]  NominalFrequency=60  UnbalancedPower=off  ActivePower=57.36e6  InductivePower=0  CapacitivePower=4.68e6  Pabc=[10e3 9e3 11e3]  QLabc=[100 90 110]  QCabc=[100 90 110]  Pabcp=[10e3 9e3 11e3]  QLabcp=[100 90 110]  QCabcp=[100 90 110]  Measurements=None  LoadType=constant PQ
  Three-Phase Series RLC Load3 : powerlib/Elements/Three-Phase Series RLC Load  LConnTagsString=A|B|C  Configuration=Y (grounded)  NominalVoltage=(230000)*0.931217  Vabc=[1e3 1e3 1e3]  Vabcp=[1e3 1e3 1e3]  NominalFrequency=60  UnbalancedPower=off  ActivePower=9.12e6  InductivePower=1.92e6  CapacitivePower=0  Pabc=[10e3 9e3 11e3]  QLabc=[100 90 110]  QCabc=[100 90 110]  Pabcp=[10e3 9e3 11e3]  QLabcp=[100 90 110]  QCabcp=[100 90 110]  Measurements=None  LoadType=constant PQ
  Three-Phase Series RLC Load4 : powerlib/Elements/Three-Phase Series RLC Load  LConnTagsString=A|B|C  Configuration=Y (grounded)  NominalVoltage=(230000)*0.942548  Vabc=[1e3 1e3 1e3]  Vabcp=[1e3 1e3 1e3]  NominalFrequency=60  UnbalancedPower=off  ActivePower=13.44e6  InductivePower=9e6  CapacitivePower=0  Pabc=[10e3 9e3 11e3]  QLabc=[100 90 110]  QCabc=[100 90 110]  Pabcp=[10e3 9e3 11e3]  QLabcp=[100 90 110]  QCabcp=[100 90 110]  Measurements=None  LoadType=constant PQ
  Three-Phase Series RLC Load5 : powerlib/Elements/Three-Phase Series RLC Load  LConnTagsString=A|B|C  Configuration=Y (grounded)  NominalVoltage=(230000)*0.942502  Vabc=[1e3 1e3 1e3]  Vabcp=[1e3 1e3 1e3]  NominalFrequency=60  UnbalancedPower=off  ActivePower=10.8e6  InductivePower=6.96e6  CapacitivePower=0  Pabc=[10e3 9e3 11e3]  QLabc=[100 90 110]  QCabc=[100 90 110]  Pabcp=[10e3 9e3 11e3]  QLabcp=[100 90 110]  QCabcp=[100 90 110]  Measurements=None  LoadType=constant PQ
  Three-Phase Series RLC Load6 : powerlib/Elements/Three-Phase Series RLC Load  LConnTagsString=A|B|C  Configuration=Y (grounded)  NominalVoltage=(230000)*0.942338  Vabc=[1e3 1e3 1e3]  Vabcp=[1e3 1e3 1e3]  NominalFrequency=60  UnbalancedPower=off  ActivePower=4.2e6  InductivePower=2.16e6  CapacitivePower=0  Pabc=[10e3 9e3 11e3]  QLabc=[100 90 110]  QCabc=[100 90 110]  Pabcp=[10e3 9e3 11e3]  QLabcp=[100 90 110]  QCabcp=[100 90 110]  Measurements=None  LoadType=constant PQ
  Three-Phase Series RLC Load7 : powerlib/Elements/Three-Phase Series RLC Load  LConnTagsString=A|B|C  Configuration=Y (grounded)  NominalVoltage=(230000)*0.941818  Vabc=[1e3 1e3 1e3]  Vabcp=[1e3 1e3 1e3]  NominalFrequency=60  UnbalancedPower=off  ActivePower=7.32e6  InductivePower=1.92e6  CapacitivePower=0  Pabc=[10e3 9e3 11e3]  QLabc=[100 90 110]  QCabc=[100 90 110]  Pabcp=[10e3 9e3 11e3]  QLabcp=[100 90 110]  QCabcp=[100 90 110]  Measurements=None  LoadType=constant PQ
  Three-Phase Series RLC Load8 : powerlib/Elements/Three-Phase Series RLC Load  LConnTagsString=A|B|C  Configuration=Y (grounded)  NominalVoltage=(230000)*0.941642  Vabc=[1e3 1e3 1e3]  Vabcp=[1e3 1e3 1e3]  NominalFrequency=60  UnbalancedPower=off  ActivePower=16.2e6  InductivePower=6.96e6  CapacitivePower=0  Pabc=[10e3 9e3 11e3]  QLabc=[100 90 110]  QCabc=[100 90 110]  Pabcp=[10e3 9e3 11e3]  QLabcp=[100 90 110]  QCabcp=[100 90 110]  Measurements=None  LoadType=constant PQ
  Three-Phase Series RLC Load9 : powerlib/Elements/Three-Phase Series RLC Load  LConnTagsString=A|B|C  Configuration=Y (grounded)  NominalVoltage=(230000)*0.941422  Vabc=[1e3 1e3 1e3]  Vabcp=[1e3 1e3 1e3]  NominalFrequency=60  UnbalancedPower=off  ActivePower=17.88e6  InductivePower=6e6  CapacitivePower=0  Pabc=[10e3 9e3 11e3]  QLabc=[100 90 110]  QCabc=[100 90 110]  Pabcp=[10e3 9e3 11e3]  QLabcp=[100 90 110]  QCabcp=[100 90 110]  Measurements=None  LoadType=constant PQ
  powergui : powerlib/powergui  Priority=1  SimulationMode=Discrete  SampleTime=50e-6  frequency=60  Iterations=50  frequencyindice=60  Pbase=120e6  ErrMax=0.0001  UnitsV=kV  UnitsW=MW  buscounter=0  FunctionMessages=off  echomessages=off  EnableUseOfTLC=off  CurrentSourceSwitches=off  DisableSnubberDevices=off  DisableRonSwitches=off  DisableVfSwitches=off  DisplayEquations=off  AutomaticDiscreteSolvers=off  SolverType=Tustin/Backward Euler (TBE)  Interpol=off  ExternalGateDelay=off  methode=off  Ts=100  x0status=blocks  SPID=on  SwTol=0  HookPort=off  NonlinearTolerance=1e-4  nMaxIteration=100  ContinueOnMaxIteration=off  RestoreLinks=warning  ResistiveCurrentMeasurement=off  Frange=[0:2:500]  Ylog=off  Xlog=on  ShowGrid=off  save=off  variable=ZData  structure=0  ZoomFFT=off  StartTime=0.0  cycles=1  DisplayStyle=1  fundamental=60  FreqAxis=off  MaxFrequency=1000  frequencyindicesteady=1  RmsSteady=1  display=off
  A : PMIOPort  Side=Right
  B : PMIOPort  Port=2  Side=Right
  C : PMIOPort  Port=3  Side=Right
  wires:
  RMS/1 -> Scope1/1
  [VB_5] -> RMS/1, Scope/1
  connections:
  Line 2-3/RConn3 -- Bus_3/RConn3
  Three-Phase Series RLC Load10/LConn1 -- Bus_9/RConn12
  Line 2-3/RConn1 -- Bus_3/RConn1
  Line 2-3/RConn2 -- Bus_3/RConn2
  Bus_7/LConn2 -- Line 4_7/LConn2
  Line 6_12/RConn3 -- Bus_6/RConn3
  Three-Phase Series RLC Load10/LConn3 -- Bus_9/RConn10
  Three-Phase Series RLC Load1/LConn2 -- Bus_3/RConn5
  Line 4_9/LConn2 -- Bus_9/RConn5
  Synchronous condensor_2/RConn3 -- 147.66/230kV/LConn3
  Three-Phase Series RLC Load/LConn1 -- Bus_2/RConn1
  Line 7-8/LConn2 -- Bus_7/RConn5
  Three-Phase Series RLC Load1/LConn1 -- Bus_3/RConn4
  Line 13-14/LConn2 -- Bus_13/RConn8
  150.42/230kV/RConn2 -- Bus_8/RConn2
  Three-Phase Series RLC Load5/LConn1 -- Bus_10/LConn1
  Three-Phase Series RLC Load/LConn2 -- Bus_2/RConn2
  Generator 1/RConn2 -- 146.28/230kV/LConn2
  Line 4_9/LConn3 -- Bus_9/RConn6
  Line 12-13/LConn2 -- Bus_12/RConn5
  Line 12-13/RConn2 -- Bus_13/RConn2
  Line 4_9/RConn3 -- Bus_4/LConn3
  Three-Phase Series RLC Load6/LConn1 -- Bus_11/LConn1
  Three-Phase Series RLC Load7/LConn2 -- Bus_12/LConn2
  Three-Phase Series RLC Load3/LConn2 -- Bus_5/LConn2
  Three-Phase Series RLC Load7/LConn3 -- Bus_12/LConn3
  Line 12-13/LConn1 -- Bus_12/RConn6
  Line 4_7/LConn3 -- Bus_7/LConn3
  Three-Phase Series RLC Load5/LConn3 -- Bus_10/LConn3
  Line 9_14/LConn1 -- Bus_14/RConn4
  Line 9-10/RConn3 -- Bus_9/RConn3
  Bus_13/RConn5 -- Line 6_13/LConn2
  Line 9-10/RConn1 -- Bus_9/RConn1
  Bus_2/RConn8 -- Line 2-3/LConn2
  Line 1-5/RConn3 -- Bus_5/RConn3
  Bus_14/RConn2 -- Line 13-14/RConn2
  150.42/230kV/RConn3 -- Bus_8/RConn3
  Synchronous condensor_3/RConn2 -- 150.42/230kV/LConn2
  Synchronous condensor_3/RConn1 -- 150.42/230kV/LConn1
  Line 1_2/LConn2 -- Bus_1/RConn2 -- B/RConn1
  Line 12-13/RConn3 -- Bus_13/RConn3
  Bus_6/LConn4 -- Line 5_6/LConn1
  Line 6_13/RConn2 -- Bus_6/RConn5
  Line 10-11/LConn2 -- Bus_11/RConn5
  Line 13-14/RConn1 -- Bus_14/RConn1
  Three-Phase Series RLC Load6/LConn2 -- Bus_11/LConn2
  Line 2-5/RConn2 -- Bus_5/RConn5
  Bus_2/RConn6 -- 144.21/230kV/RConn3
  Line 7_9/RConn3 -- Bus_7/RConn3
  " "/LConn2 -- Bus_9/LConn5
  Three-Phase Series RLC Load8/LConn2 -- Bus_13/LConn2
  Synchronous condensor_3/RConn3 -- 150.42/230kV/LConn3
  Bus_8/LConn3 -- Line 7-8/RConn3
  Line 7-8/LConn1 -- Bus_7/RConn4
  Line 5_6/RConn3 -- Bus_5/LConn6
  Three-Phase Series RLC Load9/LConn3 -- Bus_14/LConn3
  Bus_8/LConn2 -- Line 7-8/RConn2
  Line 4_7/RConn3 -- Bus_4/LConn6
  Bus_13/RConn6 -- Line 6_13/LConn3
  Line 9-10/LConn3 -- Bus_10/RConn4
  Line 4_7/RConn2 -- Bus_4/LConn5
  Line 4_7/LConn1 -- Bus_7/LConn1
  Line 9-10/RConn2 -- Bus_9/RConn2
  Line 7_9/LConn1 -- Bus_9/RConn7
  Line 7_9/RConn2 -- Bus_7/RConn2
  Bus_12/RConn2 -- Line 6_12/LConn2
  Bus_8/LConn1 -- Line 7-8/RConn1
  Line 1_2/RConn2 -- Bus_2/LConn2
  Line 7_9/RConn1 -- Bus_7/RConn1
  Line 9_14/LConn3 -- Bus_14/RConn6
  Line 6-11/LConn3 -- Bus_6/RConn9
  Line 4_9/LConn1 -- Bus_9/RConn4
  " "/LConn1 -- Bus_9/LConn4
  Line 1-5/LConn1 -- Bus_1/RConn6
  Line 9-10/LConn1 -- Bus_10/RConn6
  Three-Phase Series RLC Load10/LConn2 -- Bus_9/RConn11
  Line 9_14/RConn2 -- Bus_9/LConn2
  Line 10-11/RConn3 -- Bus_10/RConn3
  Line 7-8/LConn3 -- Bus_7/RConn6
  Line 10-11/LConn3 -- Bus_11/RConn4
  Line 4_9/RConn1 -- Bus_4/LConn1
  Line 4-5/RConn2 -- Bus_4/RConn2
  Line 10-11/LConn1 -- Bus_11/RConn6
  Line 4_9/RConn2 -- Bus_4/LConn2
  Line 6-11/RConn2 -- Bus_11/RConn2
  Three-Phase Series RLC Load2/LConn1 -- Bus_4/RConn10
  147.66/230kV/RConn3 -- Bus_6/LConn3
  Line 1_2/RConn3 -- Bus_2/LConn3
  Bus_9/LConn3 -- Line 9_14/RConn3
  Line 6-11/LConn1 -- Bus_6/RConn7
  Line 4-5/LConn2 -- Bus_5/RConn8
  Line 2-5/LConn3 -- Bus_2/LConn4
  Bus_9/LConn1 -- Line 9_14/RConn1
  Bus_4/RConn8 -- Line 3_4/LConn2
  Line 9_14/LConn2 -- Bus_14/RConn5
  Bus_4/RConn9 -- Line 3_4/LConn3
  Line 4-5/LConn3 -- Bus_5/RConn7
  146.28/230kV/LConn1 -- Generator 1/RConn1
  Bus_12/RConn3 -- Line 6_12/LConn3
  Three-Phase Series RLC Load4/LConn1 -- Bus_6/RConn10
  Line 2-5/RConn1 -- Bus_5/RConn6
  Bus_2/RConn5 -- 144.21/230kV/RConn2
  Line 7_9/LConn3 -- Bus_9/RConn9
  Bus_4/RConn7 -- Line 3_4/LConn1
  Line 1_2/LConn1 -- A/RConn1 -- Bus_1/RConn1
  Three-Phase Series RLC Load5/LConn2 -- Bus_10/LConn2
  Line 1-5/RConn2 -- Bus_5/RConn2
  Line 12-13/LConn3 -- Bus_12/RConn4
  Bus_2/LConn5 -- Line 2-5/LConn2
  Three-Phase Series RLC Load1/LConn3 -- Bus_3/RConn6
  147.66/230kV/RConn2 -- Bus_6/LConn2
  Line 2-4/LConn3 -- Bus_2/LConn9
  Line 3_4/RConn3 -- Bus_3/LConn3
  Line 2-4/RConn2 -- Bus_4/RConn5
  146.28/230kV/RConn2 -- Bus_1/LConn2
  " "/LConn3 -- Bus_9/LConn6
  Generator 2/RConn2 -- 144.21/230kV/LConn2
  Line 2-5/RConn3 -- Bus_5/RConn4
  Three-Phase Series RLC Load3/LConn3 -- Bus_5/LConn1
  Bus_3/RConn9 -- 139.38/230kV/RConn3
  Line 1_2/RConn1 -- Bus_2/LConn1
  Line 2-4/LConn2 -- Bus_2/LConn8
  Line 1-5/RConn1 -- Bus_5/RConn1
  Bus_8/RConn1 -- 150.42/230kV/RConn1
  Three-Phase Series RLC Load8/LConn1 -- Bus_13/LConn1
  Bus_2/RConn7 -- Line 2-3/LConn3
  Bus_12/RConn1 -- Line 6_12/LConn1
  Three-Phase Series RLC Load9/LConn1 -- Bus_14/LConn1
  Line 6_13/RConn1 -- Bus_6/RConn4
  Three-Phase Series RLC Load3/LConn1 -- Bus_5/LConn3
  Synchronous condensor_1/RConn2 -- 139.38/230kV/LConn2
  Line 3_4/RConn1 -- Bus_3/LConn1
  Three-Phase Series RLC Load9/LConn2 -- Bus_14/LConn2
  Line 6_12/RConn2 -- Bus_6/RConn2
  Three-Phase Series RLC Load/LConn3 -- Bus_2/RConn3
  Line 10-11/RConn1 -- Bus_10/RConn1
  147.66/230kV/RConn1 -- Bus_6/LConn1
  Line 6-11/RConn3 -- Bus_11/RConn3
  Line 2-4/LConn1 -- Bus_2/LConn7
  Generator 1/RConn3 -- 146.28/230kV/LConn3
  Three-Phase Series RLC Load2/LConn2 -- Bus_4/RConn11
  Bus_2/RConn9 -- Line 2-3/LConn1
  Three-Phase Series RLC Load2/LConn3 -- Bus_4/RConn12
  Line 5_6/RConn2 -- Bus_5/LConn5
  Three-Phase Series RLC Load7/LConn1 -- Bus_12/LConn1
  Bus_6/LConn6 -- Line 5_6/LConn3
  Three-Phase Series RLC Load4/LConn3 -- Bus_6/RConn12
  Line 7_9/LConn2 -- Bus_9/RConn8
  Synchronous condensor_2/RConn2 -- 147.66/230kV/LConn2
  Three-Phase Series RLC Load4/LConn2 -- Bus_6/RConn11
  146.28/230kV/RConn1 -- Bus_1/LConn3
  Bus_2/RConn4 -- 144.21/230kV/RConn1
  Line 6_12/RConn1 -- Bus_6/RConn1
  Line 10-11/RConn2 -- Bus_10/RConn2
  Line 6_13/RConn3 -- Bus_6/RConn6
  Line 5_6/RConn1 -- Bus_5/LConn4
  144.21/230kV/LConn1 -- Generator 2/RConn1
  Generator 2/RConn3 -- 144.21/230kV/LConn3
  Bus_3/RConn8 -- 139.38/230kV/RConn2
  Bus_6/LConn5 -- Line 5_6/LConn2
  Line 4-5/RConn1 -- Bus_4/RConn1
  Line 1-5/LConn2 -- Bus_1/RConn5
  Line 2-4/RConn3 -- Bus_4/RConn6
  Line 1_2/LConn3 -- C/RConn1 -- Bus_1/RConn3
  Synchronous condensor_2/RConn1 -- 147.66/230kV/LConn1
  Bus_13/RConn4 -- Line 6_13/LConn1
  Line 13-14/RConn3 -- Bus_14/RConn3
  Line 1-5/LConn3 -- Bus_1/RConn4
  Bus_3/RConn7 -- 139.38/230kV/RConn1
  Line 2-4/RConn1 -- Bus_4/RConn4
  Line 4-5/RConn3 -- Bus_4/RConn3
  146.28/230kV/RConn3 -- Bus_1/LConn1
  Line 12-13/RConn1 -- Bus_13/RConn1
  Line 2-5/LConn1 -- Bus_2/LConn6
  Line 3_4/RConn2 -- Bus_3/LConn2
  Line 9-10/LConn2 -- Bus_10/RConn5
  Line 6-11/RConn1 -- Bus_11/RConn1
  Three-Phase Series RLC Load8/LConn3 -- Bus_13/LConn3
  Line 13-14/LConn1 -- Bus_13/RConn9
  Line 6-11/LConn2 -- Bus_6/RConn8
  Line 4_7/RConn1 -- Bus_4/LConn4
  139.38/230kV/LConn1 -- Synchronous condensor_1/RConn1
  Line 13-14/LConn3 -- Bus_13/RConn7
  Line 4-5/LConn1 -- Bus_5/RConn9
  Three-Phase Series RLC Load6/LConn3 -- Bus_11/LConn3
  Synchronous condensor_1/RConn3 -- 139.38/230kV/LConn3

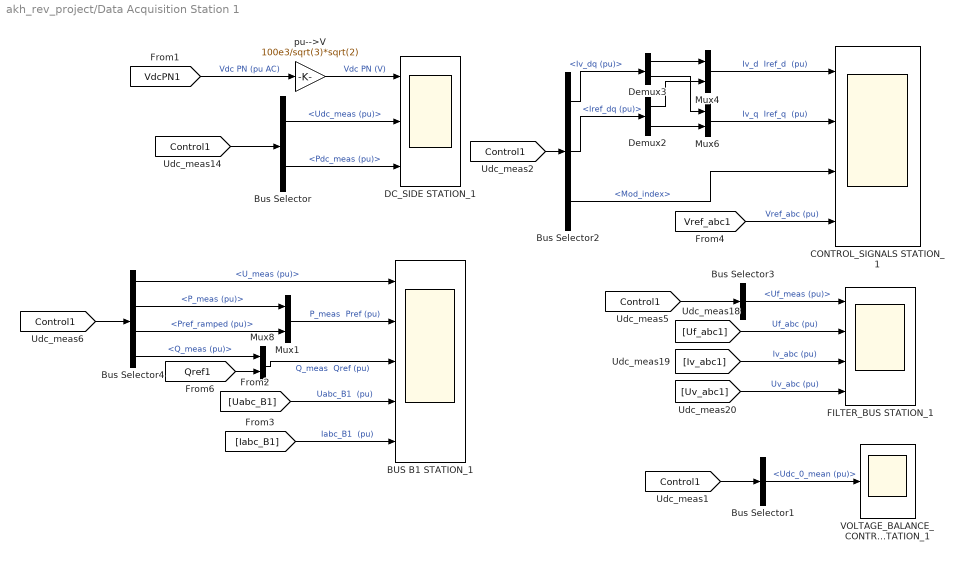
== system akh_rev_project/Data Acquisition Station 1 ==
  BUS B1 STATION_1 : Scope  NumInputPorts=5
  Bus Selector : BusSelector  OutputSignals=Udc_meas (pu),Pdc_meas (pu)
  Bus Selector1 : BusSelector  OutputSignals=Udc_0_mean (pu)
  Bus Selector2 : BusSelector  OutputSignals=Iv_dq (pu),Iref_dq (pu),Mod_index
  Bus Selector3 : BusSelector  OutputSignals=Uf_meas (pu)
  Bus Selector4 : BusSelector  OutputSignals=U_meas (pu),P_meas (pu),Pref_ramped (pu),Q_meas (pu)
  "CONTROL_SIGNALS STATION_1 " : Scope  NumInputPorts=4
  DC_SIDE STATION_1 : Scope  NumInputPorts=3
  Demux2 : Demux  Outputs=2
  Demux3 : Demux  Outputs=2
  FILTER_BUS STATION_1 : Scope  NumInputPorts=4
  Mux{1,4,6,8} (4 alike) : Mux  Inputs=2
  VOLTAGE_BALANCE_CONTROL STATION_1 : Scope
  pu-->V : Gain  Gain=100e3/sqrt(3)*sqrt(2)
  wires:
  [VdcPN1] -> pu-->V/1  "Vdc PN (pu AC)"
  Demux3/1 -> Mux4/1
  Demux2/1 -> Mux4/2
  Demux3/2 -> Mux6/1
  Demux2/2 -> Mux6/2
  [Uv_abc1] -> FILTER_BUS STATION_1/4  "Uv_abc (pu)"
  [Iv_abc1] -> FILTER_BUS STATION_1/3  "Iv_abc (pu)"
  [Uf_abc1] -> FILTER_BUS STATION_1/2  "Uf_abc (pu)"
  Bus Selector3/1 -> FILTER_BUS STATION_1/1  "<Uf_meas (pu)>"
  Bus Selector/2 -> DC_SIDE STATION_1/3  "<Pdc_meas (pu)>"
  [Control1] -> Bus Selector/1
  Bus Selector/1 -> DC_SIDE STATION_1/2  "<Udc_meas (pu)>"
  Bus Selector4/1 -> BUS B1 STATION_1/1  "<U_meas (pu)>"
  Bus Selector4/2 -> Mux1/1  "<P_meas (pu)>"
  Bus Selector4/3 -> Mux1/2  "<Pref_ramped (pu)>"
  Bus Selector4/4 -> Mux8/1  "<Q_meas (pu)>"
  [Uabc_B1] -> BUS B1 STATION_1/4  "Uabc_B1  (pu)"
  [Iabc_B1] -> BUS B1 STATION_1/5  "Iabc_B1  (pu)"
  Mux1/1 -> BUS B1 STATION_1/2  "P_meas  Pref (pu)"
  Mux8/1 -> BUS B1 STATION_1/3  "Q_meas  Qref (pu)"
  [Control1] -> Bus Selector2/1
  pu-->V/1 -> DC_SIDE STATION_1/1  "Vdc PN (V)"
  Bus Selector2/1 -> Demux3/1  "<Iv_dq (pu)>"
  Bus Selector2/3 -> "CONTROL_SIGNALS STATION_1 "/3  "<Mod_index>"
  [Control1] -> Bus Selector3/1
  [Control1] -> Bus Selector4/1
  Bus Selector2/2 -> Demux2/1  "<Iref_dq (pu)>"
  [Control1] -> Bus Selector1/1
  Bus Selector1/1 -> VOLTAGE_BALANCE_CONTROL STATION_1/1  "<Udc_0_mean (pu)>"
  Mux4/1 -> "CONTROL_SIGNALS STATION_1 "/1  "Iv_d  Iref_d  (pu)"
  Mux6/1 -> "CONTROL_SIGNALS STATION_1 "/2  "Iv_q  Iref_q  (pu)"
  [Vref_abc1] -> "CONTROL_SIGNALS STATION_1 "/4  "Vref_abc (pu)"
  [Qref1] -> Mux8/2

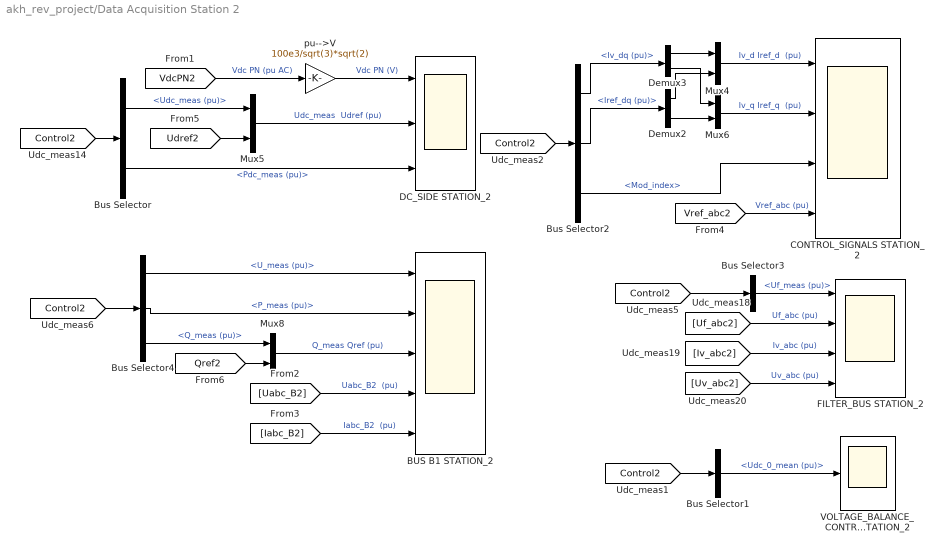
== system akh_rev_project/Data Acquisition Station 2 ==
  BUS B1 STATION_2 : Scope  NumInputPorts=5
  Bus Selector : BusSelector  OutputSignals=Udc_meas (pu),Pdc_meas (pu)
  Bus Selector1 : BusSelector  OutputSignals=Udc_0_mean (pu)
  Bus Selector2 : BusSelector  OutputSignals=Iv_dq (pu),Iref_dq (pu),Mod_index
  Bus Selector3 : BusSelector  OutputSignals=Uf_meas (pu)
  Bus Selector4 : BusSelector  OutputSignals=U_meas (pu),P_meas (pu),Q_meas (pu)
  "CONTROL_SIGNALS STATION_2 " : Scope  NumInputPorts=4
  DC_SIDE STATION_2 : Scope  NumInputPorts=3
  Demux2 : Demux  Outputs=2
  Demux3 : Demux  Outputs=2
  FILTER_BUS STATION_2 : Scope  NumInputPorts=4
  Mux{4..6,8} (4 alike) : Mux  Inputs=2
  VOLTAGE_BALANCE_CONTROL STATION_2 : Scope
  pu-->V : Gain  Gain=100e3/sqrt(3)*sqrt(2)
  wires:
  [Qref2] -> Mux8/2
  [Udref2] -> Mux5/2
  [Vref_abc2] -> "CONTROL_SIGNALS STATION_2 "/4  "Vref_abc (pu)"
  Mux6/1 -> "CONTROL_SIGNALS STATION_2 "/2  "Iv_q Iref_q  (pu)"
  Mux4/1 -> "CONTROL_SIGNALS STATION_2 "/1  "Iv_d Iref_d  (pu)"
  Bus Selector1/1 -> VOLTAGE_BALANCE_CONTROL STATION_2/1  "<Udc_0_mean (pu)>"
  [Control2] -> Bus Selector1/1
  Bus Selector2/2 -> Demux2/1  "<Iref_dq (pu)>"
  [Control2] -> Bus Selector4/1
  [Control2] -> Bus Selector3/1
  Bus Selector2/3 -> "CONTROL_SIGNALS STATION_2 "/3  "<Mod_index>"
  Bus Selector2/1 -> Demux3/1  "<Iv_dq (pu)>"
  pu-->V/1 -> DC_SIDE STATION_2/1  "Vdc PN (V)"
  [Control2] -> Bus Selector2/1
  Mux8/1 -> BUS B1 STATION_2/3  "Q_meas Qref (pu)"
  [Iabc_B2] -> BUS B1 STATION_2/5  "Iabc_B2  (pu)"
  [Uabc_B2] -> BUS B1 STATION_2/4  "Uabc_B2  (pu)"
  Bus Selector4/3 -> Mux8/1  "<Q_meas (pu)>"
  Bus Selector4/1 -> BUS B1 STATION_2/1  "<U_meas (pu)>"
  Bus Selector/1 -> Mux5/1  "<Udc_meas (pu)>"
  [Control2] -> Bus Selector/1
  Bus Selector/2 -> DC_SIDE STATION_2/3  "<Pdc_meas (pu)>"
  Bus Selector3/1 -> FILTER_BUS STATION_2/1  "<Uf_meas (pu)>"
  [Uf_abc2] -> FILTER_BUS STATION_2/2  "Uf_abc (pu)"
  [Iv_abc2] -> FILTER_BUS STATION_2/3  "Iv_abc (pu)"
  [Uv_abc2] -> FILTER_BUS STATION_2/4  "Uv_abc (pu)"
  Demux2/2 -> Mux6/2
  Demux3/2 -> Mux6/1
  Demux2/1 -> Mux4/2
  Demux3/1 -> Mux4/1
  [VdcPN2] -> pu-->V/1  "Vdc PN (pu AC)"
  Mux5/1 -> DC_SIDE STATION_2/2  "Udc_meas  Udref (pu)"
  Bus Selector4/2 -> BUS B1 STATION_2/2  "<P_meas (pu)>"

== system akh_rev_project/More info ==
